simulink model "plant"  (R2025a)
settings: Solver=FixedStepAuto  StartTime=0.0  StopTime=30  FixedStep=0.01  RelTol=1e-3
values from neighbouring files (symbols this model uses):
  b = 2    [07_july_1752.mat]    (also in 08_july.mat; spring_mass_damper.m = b_est)
  k = 16    [07_july_1752.mat]    (also in 08_july.mat = 701; spring_mass_damper.m = k_est)
  m = 1    [07_july_1752.mat]    (also in 08_july.mat; spring_mass_damper.m = m_est)
libraries: simulink x1
settings Model: Creator=ela22cbc  LastModifiedBy=ela22cbc

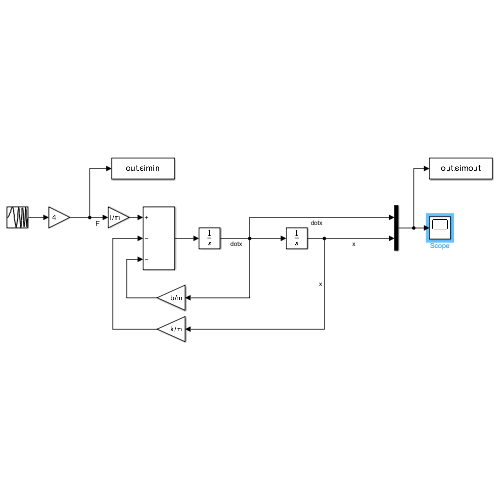
[thumbnail: Simulink's stored preview of the top-level diagram]
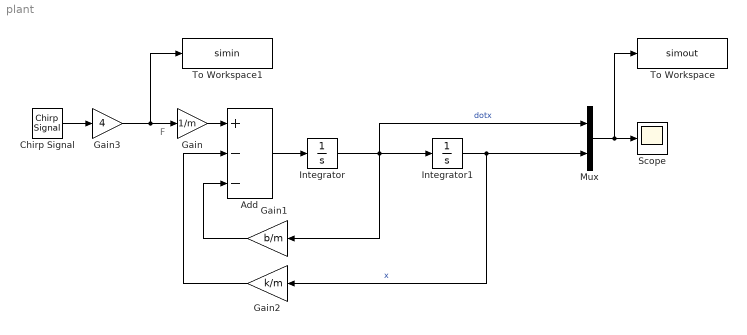
== system plant ==
  note: F
  Add : Sum  Inputs=+--
  Chirp Signal : simulink/Sources/Chirp Signal  f1=chirp_f_start  T=10  f2=chirp_f_target
  Gain : Gain  Gain=1/m
  Gain1 : Gain  Gain=b/m
  Gain2 : Gain  Gain=k/m
  Gain3 : Gain  Gain=4
  Integrator : Integrator
  Integrator1 : Integrator
  Mux : Mux  Inputs=2
  Scope : Scope
      settings: ActiveDisplayYMinimum=-0.62593187905071124  ActiveDisplayYMaximum=0.67903638831486124
  To Workspace : ToWorkspace  VariableName=simout  SampleTime=-1
  To Workspace1 : ToWorkspace  VariableName=simin  SampleTime=-1
  wires:
  Chirp Signal/1 -> Gain3/1
  Gain/1 -> Add/1
  Gain1/1 -> Add/3
  Gain2/1 -> Add/2
  Add/1 -> Integrator/1
  Integrator/1 -> Mux/1, Integrator1/1, Gain1/1  "dotx"
  Integrator1/1 -> Mux/2, Gain2/1  "x"
  Mux/1 -> To Workspace/1, Scope/1
  Gain3/1 -> To Workspace1/1, Gain/1
